simulink model "master_1"  (R2018b)
settings: Solver=VariableStepAuto  StartTime=0.0  StopTime=10.0  RelTol=1e-3
values from neighbouring files (symbols this model uses):
  Lf = 2.56    [makeBikeModel.m]    (also in makePlants.m; tunePIDs.m = 0.55)
  Lr = 1.02    [makeBikeModel.m]    (also in makePlants.m; tunePIDs.m = 0.525)
libraries: autolibshared x1
settings Model: Creator=101091775  LastModifiedBy=101091775

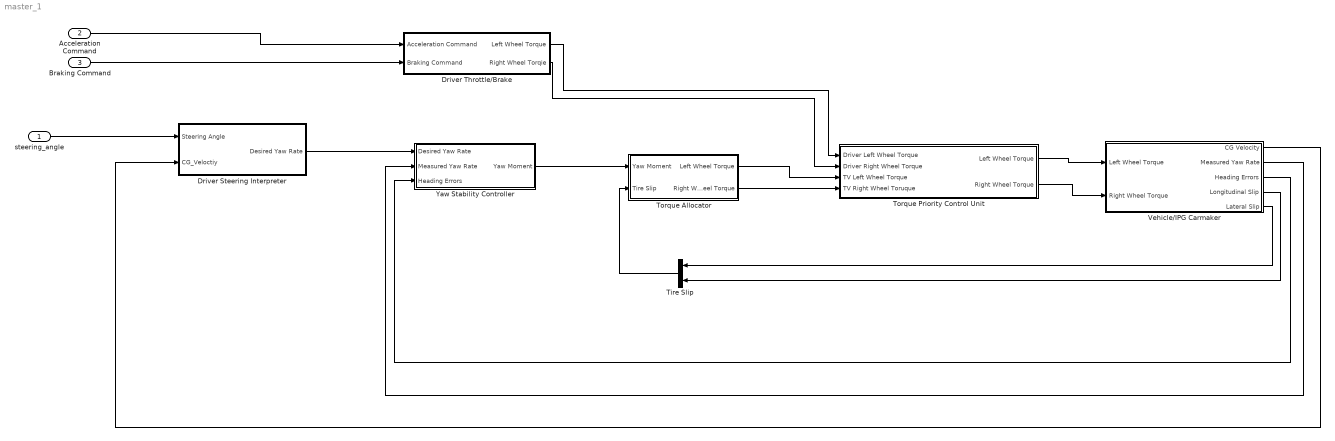
== system master_1 ==
  steering_angle : Inport
  Acceleration Command : Inport  Port=2
  Braking Command : Inport  Port=3
  " Driver Throttle/Brake" : Subsystem
  Driver Steering Interpreter : Subsystem
  Tire Slip : Concatenate
  Torque Allocator : Subsystem
  Torque Priority Control Unit : Subsystem
  Vehicle/IPG Carmaker : Subsystem
  Yaw Stability Controller : Subsystem
  wires:
  steering_angle/1 -> Driver Steering Interpreter/1(Steering Angle)
  Driver Steering Interpreter/1(Desired Yaw Rate) -> Yaw Stability Controller/1(Desired Yaw Rate)
  Yaw Stability Controller/1(Yaw Moment) -> Torque Allocator/1(Yaw Moment)
  Torque Priority Control Unit/1(Left Wheel Torque) -> Vehicle/IPG Carmaker/1(Left Wheel Torque)
  Torque Priority Control Unit/2(Right Wheel Torque) -> Vehicle/IPG Carmaker/2(Right Wheel Torque)
  Torque Allocator/2(Right Wheel Torque) -> Torque Priority Control Unit/4(TV Right Wheel Toruque)
  Torque Allocator/1(Left Wheel Torque) -> Torque Priority Control Unit/3(TV Left Wheel Torque)
  Acceleration Command/1 -> " Driver Throttle/Brake"/1(Acceleration Command)
  Braking Command/1 -> " Driver Throttle/Brake"/2(Braking Command)
  " Driver Throttle/Brake"/2(Right Wheel Torqie) -> Torque Priority Control Unit/2(Driver Right Wheel Torque)
  " Driver Throttle/Brake"/1(Left Wheel Torque) -> Torque Priority Control Unit/1(Driver Left Wheel Torque)
  Vehicle/IPG Carmaker/5(Lateral Slip) -> Tire Slip/1
  Vehicle/IPG Carmaker/4(Longitudinal Slip) -> Tire Slip/2
  Tire Slip/1 -> Torque Allocator/2(Tire Slip)
  Vehicle/IPG Carmaker/3(Heading Errors) -> Yaw Stability Controller/3(Heading Errors)
  Vehicle/IPG Carmaker/2(Measured Yaw Rate) -> Yaw Stability Controller/2(Measured Yaw Rate)
  Vehicle/IPG Carmaker/1(CG Velocity) -> Driver Steering Interpreter/2(CG_Veloctiy)

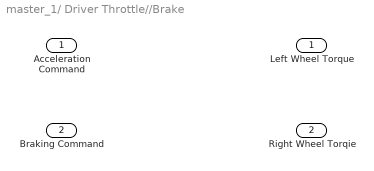
== system master_1/ Driver Throttle//Brake ==
  Acceleration Command : Inport
  Braking Command : Inport  Port=2
  Left Wheel Torque : Outport
  Right Wheel Torqie : Outport  Port=2

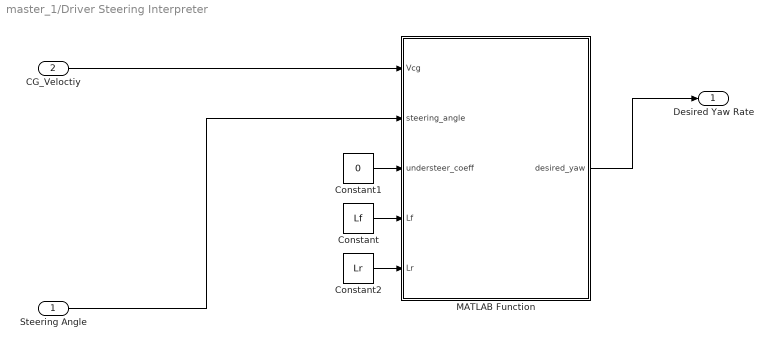
== system master_1/Driver Steering Interpreter ==
  Steering Angle : Inport
  CG_Veloctiy : Inport  Port=2
  Constant : Constant  Value=Lf
  Constant1 : Constant  Value=0
  Constant2 : Constant  Value=Lr
  MATLAB Function : MATLAB Function  TreatAsAtomicUnit=on
  Desired Yaw Rate : Outport
  wires:
  Constant/1 -> MATLAB Function/4(Lf)
  Constant2/1 -> MATLAB Function/5(Lr)
  CG_Veloctiy/1 -> MATLAB Function/1(Vcg)
  MATLAB Function/1(desired_yaw) -> Desired Yaw Rate/1
  Steering Angle/1 -> MATLAB Function/2(steering_angle)
  Constant1/1 -> MATLAB Function/3(understeer_coeff)

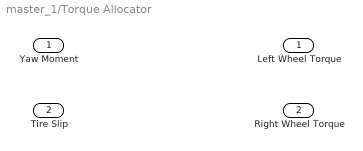
== system master_1/Torque Allocator ==
  Yaw Moment : Inport
  Tire Slip : Inport  Port=2
  Left Wheel Torque : Outport
  Right Wheel Torque : Outport  Port=2

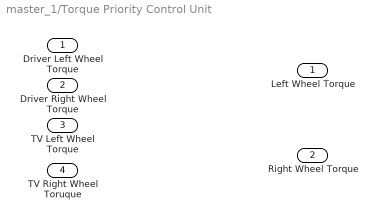
== system master_1/Torque Priority Control Unit ==
  Driver Left Wheel Torque : Inport
  Driver Right Wheel Torque : Inport  Port=2
  TV Left Wheel Torque : Inport  Port=3
  TV Right Wheel Toruque : Inport  Port=4
  Left Wheel Torque : Outport
  Right Wheel Torque : Outport  Port=2

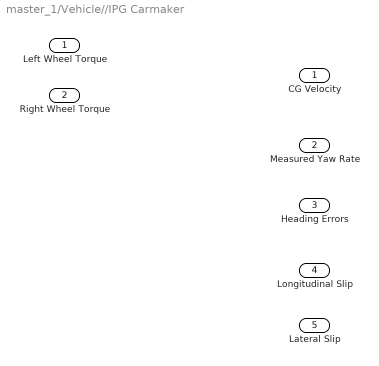
== system master_1/Vehicle//IPG Carmaker ==
  Left Wheel Torque : Inport
  Right Wheel Torque : Inport  Port=2
  CG Velocity : Outport
  Measured Yaw Rate : Outport  Port=2
  Heading Errors : Outport  Port=3
  Longitudinal Slip : Outport  Port=4
  Lateral Slip : Outport  Port=5

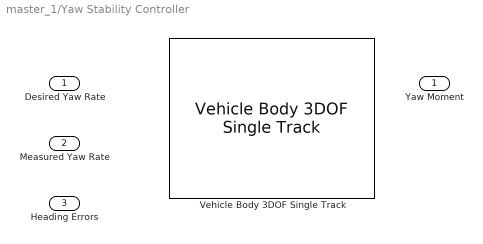
== system master_1/Yaw Stability Controller ==
  Desired Yaw Rate : Inport
  Measured Yaw Rate : Inport  Port=2
  Heading Errors : Inport  Port=3
  Vehicle Body 3DOF Single Track : autolibshared/Vehicle Body 3DOF Single Track  trackMode=Single (bicycle)  inputMode=External longitudinal velocity  frontSteerMode=on  rearSteerMode=off  windMode=off  muMode=off  extFMode=off  extMMode=off  aMode=2  NF=2  NR=2  m=2000  a=1.4  b=1.6  h=0.35  X_o=0  xdot_o=0  CalphaMode=off  sigmaMode=on  d=0  w=[1.4,1.4]  Cy_f=12e3  Cy_r=11e3  sigma_f=.1  sigma_r=.1  alpha_f_brk=[-.1 .1]  Cy_f_data=[-9e3 9e3]  alpha_r_brk=[-.1 .1]  Cy_r_data=[-9e3 9e3]  Y_o=0  ydot_o=0  Izz=4000  psi_o=0  r_o=0  Af=2  Cd=.3  Cl=.1  Cpm=.1  beta_w=[0:0.01:0.3]  Cs=[0:0.03:0.9]  Cym=[0:0.01:0.3]  Pabs=101325  Tair=273  g=9.81  mu=1  xdot_tol=.01  Fznom=5000  Fxtire_sat=7e4  Fytire_sat=7e4  longOff=0  latOff=0  vertOff=0
      settings: SourceProductName=Powertrain Blockset  SourceProductBaseCode=PW
  Yaw Moment : Outport

== matlab function master_1/Driver Steering Interpreter/MATLAB Function ==
  data: Vcg input; desired_yaw output; steering_angle input; understeer_coeff input; Lf input; Lr input
function desired_yaw = desiredYaw(Vcg , steering_angle, understeer_coeff, Lf, Lr)
desired_yaw = 0;
desired_yaw = Vcg*steering_angle/((Lf*Lr) + understeer_coeff*Vcg^2);
